simulink model "Buck_converter_step1"  (Simulink 8.4)
settings: Solver=ode23tb  StartTime=0.0  StopTime=0.01  MaxStep=1e-6  RelTol=1e-4
PreLoadFcn:
  | Ts = 2e-6
  | Tsc = 1e-7
libraries: powerlib x12
settings Model: Creator=kfukui  LastModifiedBy=kotsuka
settings DebuggingCC: FcnCallInpInsideContextMsg=EnableAllAsWarning

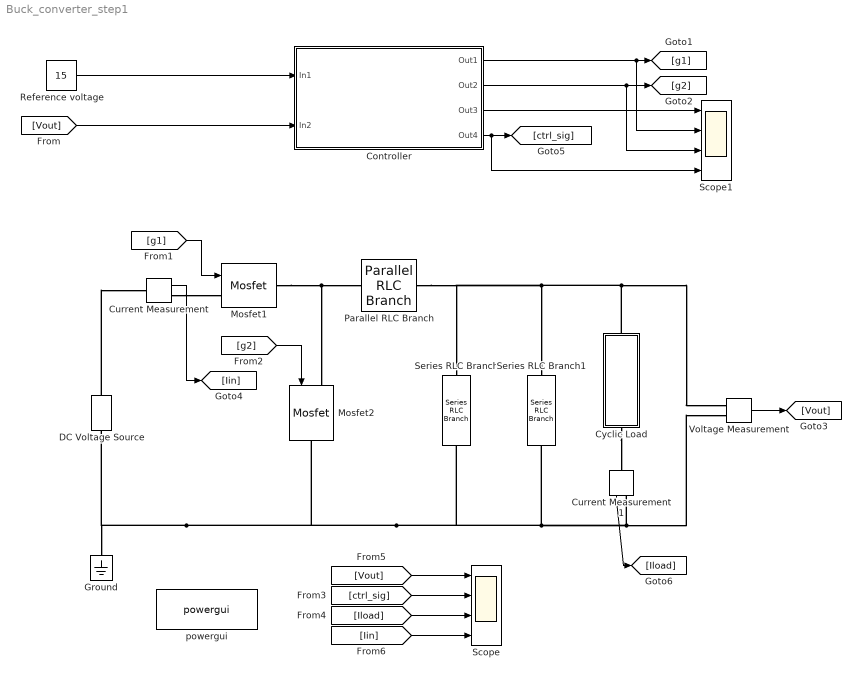
== system Buck_converter_step1 ==
  Controller : Subsystem
  Current Measurement : powerlib/Measurements/Current Measurement  PhasorSimulation=off  OutputType=Complex  PSBequivalent=0
  Current Measurement1 : powerlib/Measurements/Current Measurement  PhasorSimulation=off  OutputType=Complex  PSBequivalent=0
  Cyclic Load : Subsystem
  DC Voltage Source : powerlib/Electrical Sources/DC Voltage Source  Amplitude=30  Measurements=None
  Ground : powerlib/Elements/Ground  LConnTagsString=a
  Mosfet1 : powerlib/Power Electronics/Mosfet  Ron=0.1  Lon=0  Rd=0.01  Vfd=0.8  IC=0  Rs=1e5  Cs=inf  Measurements=off
  Mosfet2 : powerlib/Power Electronics/Mosfet  Ron=0.1  Lon=0  Rd=0.01  Vfd=0.8  IC=0  Rs=1e5  Cs=inf  Measurements=off
  Parallel RLC Branch : powerlib/Elements/Parallel RLC Branch  LConnTagsString=a  RConnTagsString=__new0  BranchType=RL  Resistance=10e3  Inductance=1e-3  SetiL0=off  InitialCurrent=0  Capacitance=1e-6  Setx0=off  InitialVoltage=0  Measurements=None
  Reference voltage : Constant  Value=15
  Scope : Scope  NumInputPorts=4
      settings: TimeRange=0.01  YMin=0~0~-1~-1  YMax=25~1~3~8
  Scope1 : Scope  NumInputPorts=4
      settings: TimeRange=0.001041229385307346  YMin=-1~0~0~-1  YMax=1~1~1~1
  Series RLC Branch : powerlib/Elements/Series RLC Branch  LConnTagsString=__new0  RConnTagsString=__new0  BranchType=C  Resistance=1  Inductance=1e-3  SetiL0=off  InitialCurrent=0  Capacitance=22e-6  Setx0=off  InitialVoltage=0  Measurements=None
  Series RLC Branch1 : powerlib/Elements/Series RLC Branch  LConnTagsString=__new0  RConnTagsString=__new0  BranchType=R  Resistance=3.75  Inductance=1e-3  SetiL0=off  InitialCurrent=0  Capacitance=22e-6  Setx0=off  InitialVoltage=0  Measurements=None
  Voltage Measurement : powerlib/Measurements/Voltage Measurement  PhasorSimulation=off  OutputType=Complex  PSBequivalent=0
  powergui : powerlib/powergui  Priority=1  SimulationMode=Continuous  SolverType=Tustin  SampleTime=50e-6  frequency=60  SPID=off  DisableSnubberDevices=off  DisableRonSwitches=off  DisableVfSwitches=off  SwTol=0  DisplayEquations=off  Interpol=off  methode=off  Ts=100  frequencyindice=0  Pbase=100e6  ErrMax=1e-4  Iterations=50  UnitsV=kV  UnitsW=MW  FunctionMessages=off  echomessages=off  HookPort=off  EnableUseOfTLC=off  x0status=blocks  RestoreLinks=warning  ResistiveCurrentMeasurement=off  Frange=[0:2:500]  Ylog=off  Xlog=on  ShowGrid=off  save=off  variable=ZData  structure=0  ZoomFFT=off  StartTime=0.0  cycles=1  DisplayStyle=1  fundamental=60  FreqAxis=off  MaxFrequency=1000  frequencyindicesteady=1  RmsSteady=1  display=off
  wires:
  Voltage Measurement/1 -> [Vout]
  Controller/1(Out1) -> [g1], Scope1/2
  Controller/2(Out2) -> [g2], Scope1/3
  [g1] -> Mosfet1/1
  [g2] -> Mosfet2/1
  Current Measurement/1 -> [Iin]
  Current Measurement1/1 -> [Iload]
  [Vout] -> Scope/1
  [ctrl_sig] -> Scope/2
  [Iload] -> Scope/3
  [Iin] -> Scope/4
  Controller/3(Out3) -> Scope1/1
  Controller/4(Out4) -> [ctrl_sig], Scope1/4
  Reference voltage/1 -> Controller/1(In1)
  [Vout] -> Controller/2(In2)
  connections:
  DC Voltage Source/RConn1 -- Current Measurement/LConn1
  Current Measurement/RConn1 -- Mosfet1/LConn1
  Mosfet1/RConn1 -- Mosfet2/LConn1 -- Parallel RLC Branch/LConn1
  Cyclic Load/LConn1 -- Parallel RLC Branch/RConn1 -- Series RLC Branch/LConn1 -- Series RLC Branch1/LConn1 -- Voltage Measurement/LConn1
  Series RLC Branch1/RConn1 -- Series RLC Branch/RConn1 -- Mosfet2/RConn1 -- DC Voltage Source/LConn1 -- Ground/LConn1 -- Current Measurement1/RConn1 -- Voltage Measurement/LConn2
  Cyclic Load/RConn1 -- Current Measurement1/LConn1

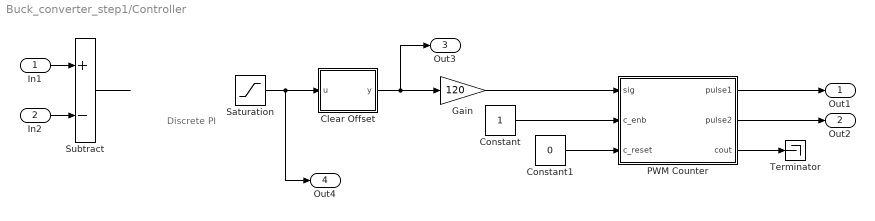
== system Buck_converter_step1/Controller ==
  note: Discrete PI
  In1 : Inport
  In2 : Inport  Port=2
  Clear Offset : MATLAB Function  TreatAsAtomicUnit=on
  Constant : Constant  SampleTime=Tsc
  Constant1 : Constant  Value=0  SampleTime=Tsc
  Gain : Gain  Gain=120
  PWM Counter : MATLAB Function  TreatAsAtomicUnit=on
  Saturation : Saturate  UpperLimit=0.95  LowerLimit=0.01
  Subtract : Sum  Inputs=+-
  Terminator : Terminator
  Out1 : Outport
  Out2 : Outport  Port=2
  Out3 : Outport  Port=3
  Out4 : Outport  Port=4
  wires:
  Clear Offset/1(y) -> Out3/1, Gain/1
  Saturation/1 -> Clear Offset/1(u), Out4/1
  ? -> Saturation/1
  Subtract/1 -> ?
  In1/1 -> Subtract/1
  In2/1 -> Subtract/2
  PWM Counter/1(pulse1) -> Out1/1
  PWM Counter/2(pulse2) -> Out2/1
  Constant/1 -> PWM Counter/2(c_enb)
  Constant1/1 -> PWM Counter/3(c_reset)
  Gain/1 -> PWM Counter/1(sig)
  PWM Counter/3(cout) -> Terminator/1

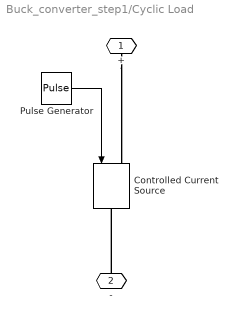
== system Buck_converter_step1/Cyclic Load ==
  Controlled Current Source : powerlib/Electrical Sources/Controlled Current Source  Initialize=on  Source_Type=AC  Amplitude=0  Phase=0  Frequency=0  Measurements=None
  Pulse Generator : DiscretePulseGenerator  PulseType=Time based  Amplitude=2  Period=1/200  PulseWidth=50  PhaseDelay=1/400
  + : PMIOPort  Port=1  Side=Left
  - : PMIOPort  Port=2  Side=Right
  wires:
  Pulse Generator/1 -> Controlled Current Source/1
  connections:
  +/RConn1 -- Controlled Current Source/LConn1
  -/RConn1 -- Controlled Current Source/RConn1

== matlab function Controller/PWM Counter ==
  data: sig input double; pulse1 output double; c_enb input double; c_reset input double; pulse2 output double; cout output double
function [pulse1,pulse2, cout] = fcn(sig, c_enb, c_reset)
%#codegen

coutmax = 124;
persistent ctmp
if isempty(ctmp)
	ctmp = 0;
end
if c_reset
	ctmp = 0;
else
	if c_enb
		if ctmp < coutmax
			ctmp = ctmp + 1;
		else
			ctmp = -125;
		end
	end
end
cout = ctmp;

if ctmp < sig
	pulse1 = 1;
	pulse2 = 0;
else
	pulse1 = 0;
	pulse2 = 1;
end

== matlab function Controller/Clear Offset ==
  data: u input double; y output double
function y = fcn(u)
%#codegen

tmp = 2*u;
y = tmp-1;
